simulink model "xe_hai_banh_cb"  (R2019a)
settings: Solver=FixedStepAuto  StartTime=0.0  StopTime=20  FixedStep=0.01  RelTol=1e-3
undefined symbols (not defined in the file): a, beta, fw, J_phi, Jm, Jw, L, M, m, n, R, W, x1_in, x2_in, x4_in, x5_in, x7_in, x8_in
settings Model: Creator=ACER  LastModifiedBy=chute

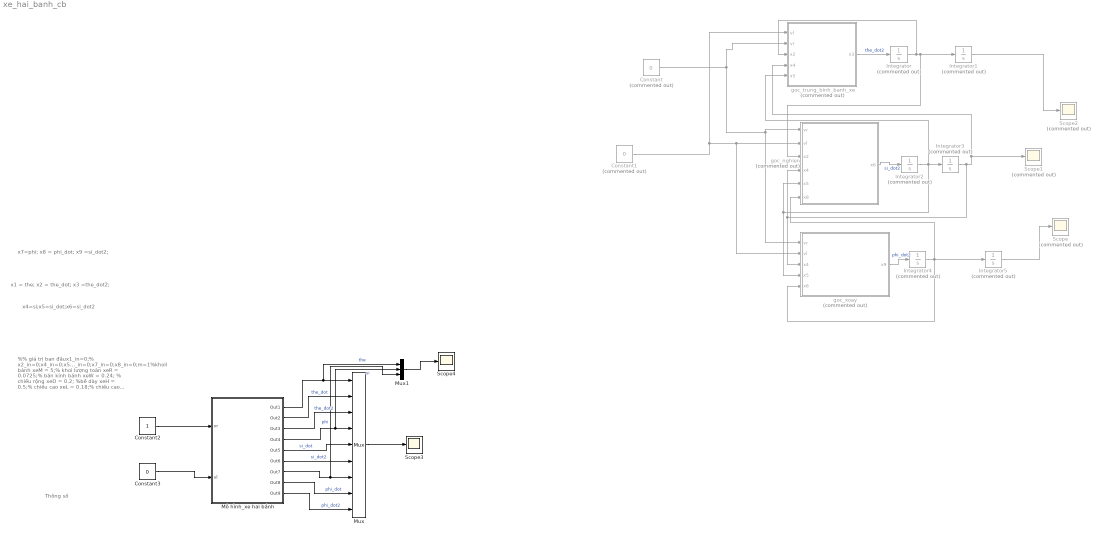
== system xe_hai_banh_cb ==
  note: x4=si;x5=si_dot;x6=si_dot2
  note: %% giá trị ban đầux1_in=0;% x2_in=0;x4_in=0;x5_in=0;x7_in=0;x8_in=0;m=1%khoil bánh xeM = 5;% khoi lượng toàn xeR = 0.0725;% bán kính bánh xeW = 0.24; % chiều rộng xeD = 0.2; %bề dày xeH = 0.5;% chiều cao xeL = 0.18;% chiều cao thân xefw = 0.18;% hệ số ma sát mặt di chuyểnfm = 0.002;% hệ số ma sát động cơJm = m*R^2/2;% momen quán tính đcJsi = M*L^2/3; % momen quan tính phần thân xeJ_phi = M*(W^2 + D^2)/12; % momen quan tinh toàn xeJw = m*R^2/2; %momen quan tinh banh xeRm = 50; % ddien trở Kb = 0.468; % hệ số dcKt = 0.317; % hệ số dcn = 40; % tỉ số truyền dcg = 9.81; %gia tóc ttbeta = (n*Kt*Kb)/Rm + fm;a=(n*Kt)/Rm;
  note: Thông số
  note: x1 = the; x2 = the_dot; x3 =the_dot2;
  note: x7=phi; x8 = phi_dot; x9 =si_dot2;
  Constant : Constant  Commented=on  Value=0
  Constant1 : Constant  Commented=on  Value=0
  Constant2 : Constant
  Constant3 : Constant  Value=0
  Integrator : Integrator  Commented=on
  Integrator1 : Integrator  Commented=on  InitialCondition=0.0012
  Integrator2 : Integrator  Commented=on
  Integrator3 : Integrator  Commented=on  InitialCondition=0.0001
  Integrator4 : Integrator  Commented=on
  Integrator5 : Integrator  Commented=on  InitialCondition=0.0001
  Mux : Mux  Inputs=9
  Mux1 : Mux  Inputs=3
  "Mô hình_xe hai bánh " : Subsystem
  Scope : Scope  Commented=on
  Scope1 : Scope  Commented=on
  Scope2 : Scope  Commented=on
  Scope3 : Scope
  Scope4 : Scope
  goc_nghien : MATLAB Function  Commented=on  TreatAsAtomicUnit=on
  goc_trung_binh_banh_xe : MATLAB Function  Commented=on  TreatAsAtomicUnit=on
  "goc_xoay " : MATLAB Function  Commented=on  TreatAsAtomicUnit=on
  wires:
  Integrator/1 -> goc_nghien/3(x2), Integrator1/1, goc_trung_binh_banh_xe/3(x2)
  Integrator4/1 -> "goc_xoay "/5(x8), Integrator5/1, goc_nghien/6(x8)
  Integrator2/1 -> goc_nghien/5(x5), "goc_xoay "/4(x5), goc_trung_binh_banh_xe/5(x5), Integrator3/1
  Integrator3/1 -> goc_nghien/4(x4), "goc_xoay "/3(x4), goc_trung_binh_banh_xe/4(x4), Scope1/1
  Constant1/1 -> goc_trung_binh_banh_xe/1(vl), "goc_xoay "/2(vl), goc_nghien/2(vl)
  goc_nghien/1(x6) -> Integrator2/1  "si_dot2"
  Constant/1 -> goc_trung_binh_banh_xe/2(vr), "goc_xoay "/1(vr), goc_nghien/1(vr)
  "goc_xoay "/1(x9) -> Integrator4/1  "phi_dot2"
  goc_trung_binh_banh_xe/1(x3) -> Integrator/1  "the_dot2"
  Integrator5/1 -> Scope/1
  Integrator1/1 -> Scope2/1
  Mux/1 -> Scope3/1
  "Mô hình_xe hai bánh "/9(Out9) -> Mux/9  "phi_dot2"
  "Mô hình_xe hai bánh "/8(Out8) -> Mux/8  "phi_dot"
  "Mô hình_xe hai bánh "/7(Out7) -> Mux1/3, Mux/7  "phi"
  "Mô hình_xe hai bánh "/6(Out6) -> Mux/6  "si_dot2"
  "Mô hình_xe hai bánh "/5(Out5) -> Mux/5  "si_dot"
  "Mô hình_xe hai bánh "/4(Out4) -> Mux1/2, Mux/4  "si"
  "Mô hình_xe hai bánh "/3(Out3) -> Mux/3  "the_dot2"
  "Mô hình_xe hai bánh "/2(Out2) -> Mux/2  "the_dot"
  "Mô hình_xe hai bánh "/1(Out1) -> Mux1/1, Mux/1  "the"
  Constant2/1 -> "Mô hình_xe hai bánh "/1("vr ")
  Constant3/1 -> "Mô hình_xe hai bánh "/2("vl ")
  Mux1/1 -> Scope4/1

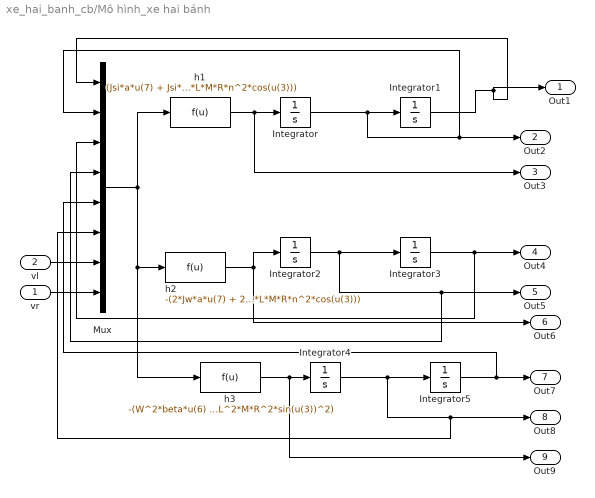
== system xe_hai_banh_cb/Mô hình_xe hai bánh  ==
  "vr " : Inport
  "vl " : Inport  Port=2
  Integrator : Integrator  InitialCondition=x2_in
  Integrator1 : Integrator  InitialCondition=x1_in
  Integrator2 : Integrator  InitialCondition=x5_in
  Integrator3 : Integrator  InitialCondition=x4_in
  Integrator4 : Integrator  InitialCondition=x8_in
  Integrator5 : Integrator  InitialCondition=x7_in
  Mux : Mux  Inputs=8
  "h1 " : Fcn  Expr=(Jsi*a*u(7) + Jsi*a*u(8) - 2*Jsi*beta*u(2) + 2*Jsi*beta*u(4) - 2*Jsi*fw*u(2) + L^2*M*a*u(7) + L^2*M*a*u(8) - 2*L^2*M*beta*u(2) + 2*L^2*M*beta*u(4) - 2*L^2*M*fw*u(2) - 4*Jm*fw*n^2*u(2) + L^3*M^2*R*u(4)^2*sin(u(3)) - 2*L*M*R*beta*u(2)*cos(u(3)) + 2*L*M*R*beta*u(4)*cos(u(3)) - L^3*M^2*R*u(6)^2*cos(u(3))^2*sin(u(3)) - L^2*M^2*R*g*cos(u(3))*sin(u(3)) + Jsi*L*M*R*u(4)^2*sin(u(3)) + 2*Jm*L*M*g*n^2*sin(u(3)) + L*M*R*a*u(7)*cos(u(3)) + L*M*R*a*u(8)*cos(u(3)) + 2*Jm*L^2*M*n^2*u(6)^2*cos(u(3))*sin(u(3)) + 2*Jm*L*M*R*n^2*u(4)^2*sin(u(3)))/(2*Jsi*Jw + L^2*M^2*R^2 + 2*Jw*L^2*M + Jsi*M*R^2 + 2*Jm*Jsi*n^2 + 4*Jm*Jw*n^2 + 2*Jsi*R^2*m + 2*Jm*L^2*M*n^2 + 2*Jm*M*R^2*n^2 + 2*L^2*M*R^2*m + 4*Jm*R^2*m*n^2 - L^2*M^2*R^2*cos(u(3))^2 + 4*Jm*L*M*R*n^2*cos(u(3)))
  "h2 " : Fcn  Expr=-(2*Jw*a*u(7) + 2*Jw*a*u(8) - 4*Jw*beta*u(2) + 4*Jw*beta*u(4) + M*R^2*a*u(7) + M*R^2*a*u(8) - 2*M*R^2*beta*u(2) + 2*M*R^2*beta*u(4) + 2*R^2*a*m*u(7) + 2*R^2*a*m*u(8) + 4*Jm*fw*n^2*u(2) - 4*R^2*beta*m*u(2) + 4*R^2*beta*m*u(4) - L*M^2*R^2*g*sin(u(3)) - 2*Jw*L*M*g*sin(u(3)) - 2*L*M*R*beta*u(2)*cos(u(3)) + 2*L*M*R*beta*u(4)*cos(u(3)) - 2*L*M*R*fw*u(2)*cos(u(3)) + L^2*M^2*R^2*u(4)^2*cos(u(3))*sin(u(3)) - L^2*M^2*R^2*u(6)^2*cos(u(3))*sin(u(3)) - 2*Jw*L^2*M*u(6)^2*cos(u(3))*sin(u(3)) - 2*Jm*L*M*g*n^2*sin(u(3)) - 2*L*M*R^2*g*m*sin(u(3)) + L*M*R*a*u(7)*cos(u(3)) + L*M*R*a*u(8)*cos(u(3)) - 2*Jm*L^2*M*n^2*u(6)^2*cos(u(3))*sin(u(3)) - 2*L^2*M*R^2*m*u(6)^2*cos(u(3))*sin(u(3)) - 2*Jm*L*M*R*n^2*u(4)^2*sin(u(3)))/(2*Jsi*Jw + L^2*M^2*R^2 + 2*Jw*L^2*M + Jsi*M*R^2 + 2*Jm*Jsi*n^2 + 4*Jm*Jw*n^2 + 2*Jsi*R^2*m + 2*Jm*L^2*M*n^2 + 2*Jm*M*R^2*n^2 + 2*L^2*M*R^2*m + 4*Jm*R^2*m*n^2 - L^2*M^2*R^2*cos(u(3))^2 + 4*Jm*L*M*R*n^2*cos(u(3)))
  "h3 " : Fcn  Expr=-(W^2*beta*u(6) + W^2*fw*u(6) + R*W*a*u(7) - R*W*a*u(8) + 4*L^2*M*R^2*u(4)*u(6)*cos(u(3))*sin(u(3)))/(2*J_phi*R^2 + Jw*W^2 + Jm*W^2*n^2 + R^2*W^2*m + 2*L^2*M*R^2*sin(u(3))^2)
  Out1 : Outport
  Out2 : Outport  Port=2
  Out3 : Outport  Port=3
  Out4 : Outport  Port=4
  Out5 : Outport  Port=5
  Out6 : Outport  Port=6
  Out7 : Outport  Port=7
  Out8 : Outport  Port=8
  Out9 : Outport  Port=9
  wires:
  Mux/1 -> "h2 "/1, "h3 "/1, "h1 "/1
  "vr "/1 -> Mux/8
  "vl "/1 -> Mux/7
  Integrator/1 -> Mux/2, Out2/1, Integrator1/1
  Integrator1/1 -> Mux/1, Out1/1
  "h2 "/1 -> Integrator2/1, Out6/1
  "h3 "/1 -> Out9/1, Integrator4/1
  Integrator4/1 -> Mux/6, Out8/1, Integrator5/1
  Integrator3/1 -> Mux/3, Out4/1
  Integrator5/1 -> Mux/5, Out7/1
  "h1 "/1 -> Out3/1, Integrator/1
  Integrator2/1 -> Mux/4, Out5/1, Integrator3/1

== matlab function xe_hai_banh_cb/goc_nghien ==
  data: vr input; x6 output; vl input; x2 input; x4 input; x5 input; x8 input
function x6= si_dot2(vr,vl,x2,x4,x5,x8)
m=1%khoil bánh xe
M = 5;% khoi lượng toàn xe
R = 0.0725;% bán kính bánh xe
W = 0.24; % chiều rộng xe
D = 0.2 %bề dày xe
H = 0.5;% chiều cao xe
L = 0.18;% chiều cao thân xe
fw = 0.18;% hệ số ma sát mặt di chuyển
fm = 0.002;% hệ số ma sát động cơ
Jm = m*R^2/2;% momen quán tính đc
Jsi = M*L^2/3; % momen quan tính phần thân xe
J_phi = M*(W^2 + D^2)/12; % momen quan tinh toàn xe
Jw = m*R^2/2; %momen quan tinh banh xe
Rm = 50; % ddien trở 
Kb = 0.468; % hệ số dc
Kt = 0.317; % hệ số dc
n = 40; % tỉ số truyền dc
g = 9.81; %gia tóc tt
beta = (n*Kt*Kb)/Rm + fm;
a=(n*Kt)/Rm;
x6= -(2*Jw*a*vl + 2*Jw*a*vr - 4*Jw*beta*x2 + ...
    4*Jw*beta*x5 + M*R^2*a*vl + M*R^2*a*vr -...
    2*M*R^2*beta*x2 + 2*M*R^2*beta*x5 + 2*R^2*a*m*vl +...
    2*R^2*a*m*vr + 4*Jm*fw*n^2*x2 - 4*R^2*beta*m*x2 +...
    4*R^2*beta*m*x5 - L*M^2*R^2*g*sin(x4) - 2*Jw*L*M*g*sin(x4) - ...
    2*L*M*R*beta*x2*cos(x4) + 2*L*M*R*beta*x5*cos(x4) - 2*L*M*R*fw*x2*cos(x4) +...
    L^2*M^2*R^2*x5^2*cos(x4)*sin(x4) - L^2*M^2*R^2*x8^2*cos(x4)*sin(x4) -...
    2*Jw*L^2*M*x8^2*cos(x4)*sin(x4) - 2*Jm*L*M*g*n^2*sin(x4) - ...
    2*L*M*R^2*g*m*sin(x4) + L*M*R*a*vl*cos(x4) + L*M*R*a*vr*cos(x4) -...
    2*Jm*L^2*M*n^2*x8^2*cos(x4)*sin(x4) - 2*L^2*M*R^2*m*x8^2*cos(x4)*sin(x4) -...
    2*Jm*L*M*R*n^2*x5^2*sin(x4))/(2*Jsi*Jw + L^2*M^2*R^2 +...
    2*Jw*L^2*M + Jsi*M*R^2 + 2*Jm*Jsi*n^2 + 4*Jm*Jw*n^2 +...
    2*Jsi*R^2*m + 2*Jm*L^2*M*n^2 + 2*Jm*M*R^2*n^2 + 2*L^2*M*R^2*m +...
    4*Jm*R^2*m*n^2 - L^2*M^2*R^2*cos(x4)^2 + 4*Jm*L*M*R*n^2*cos(x4));

== matlab function xe_hai_banh_cb/goc_trung_binh_banh_xe ==
  data: vl input; x3 output; vr input; x2 input; x4 input; x5 input
function x3 =the_dot2(vl,vr,x2,x4,x5)
m=1%khoil bánh xe
M = 5;% khoi lượng toàn xe
R = 0.0725;% bán kính bánh xe
W = 0.24; % chiều rộng xe
D = 0.2 %bề dày xe
H = 0.5;% chiều cao xe
L = 0.18;% chiều cao thân xe
fw = 0.18;% hệ số ma sát mặt di chuyển
fm = 0.002;% hệ số ma sát động cơ
Jm = m*R^2/2;% momen quán tính đc
Jsi = M*L^2/3; % momen quan tính phần thân xe
J_phi = M*(W^2 + D^2)/12; % momen quan tinh toàn xe
Jw = m*R^2/2; %momen quan tinh banh xe
Rm = 50; % ddien trở 
Kb = 0.468; % hệ số dc
Kt = 0.317; % hệ số dc
n = 40; % tỉ số truyền dc
g = 9.81; %gia tóc tt
beta = (n*Kt*Kb)/Rm + fm;
a=(n*Kt)/Rm;
 x3=(Jsi*a*vl + Jsi*a*vr - 2*Jsi*beta*x2 + 2*Jsi*beta*x5 -...
     2*Jsi*fw*x2 + L^2*M*a*vl + L^2*M*a*vr - 2*L^2*M*beta*x2 +...
     2*L^2*M*beta*x5 - 2*L^2*M*fw*x2 - 4*Jm*fw*n^2*x2 +...
     L^3*M^2*R*x5^2*sin(x4) - 2*L*M*R*beta*x2*cos(x4) + 2*L*M*R*beta*x5*cos(x4)...
     - L^3*M^2*R*x8^2*cos(x4)^2*sin(x4) - L^2*M^2*R*g*cos(x4)*sin(x4) +...
     Jsi*L*M*R*x5^2*sin(x4) + 2*Jm*L*M*g*n^2*sin(x4) + L*M*R*a*vl*cos(x4) +...
     L*M*R*a*vr*cos(x4) + 2*Jm*L^2*M*n^2*x8^2*cos(x4)*sin(x4) +...
     2*Jm*L*M*R*n^2*x5^2*sin(x4))/(2*Jsi*Jw + L^2*M^2*R^2 + 2*Jw*L^2*M +...
     Jsi*M*R^2 + 2*Jm*Jsi*n^2 + 4*Jm*Jw*n^2 + 2*Jsi*R^2*m + 2*Jm*L^2*M*n^2 +...
     2*Jm*M*R^2*n^2 + 2*L^2*M*R^2*m + 4*Jm*R^2*m*n^2 - L^2*M^2*R^2*cos(x4)^2 +...
     4*Jm*L*M*R*n^2*cos(x4));
end

== matlab function xe_hai_banh_cb/goc_xoay  ==
  data: vr input; x9 output; vl input; x4 input; x5 input; x8 input
function x9 = phi_dot2(vr,vl,x4,x5,x8)
m=1;%khoil bánh xe
M = 5;% khoi lượng toàn xe
R = 0.0725;% bán kính bánh xe
W = 0.24; % chiều rộng xe
D = 0.2 %bề dày xe
H = 0.5;% chiều cao xe
L = 0.18;% chiều cao thân xe
fw = 0.18;% hệ số ma sát mặt di chuyển
fm = 0.002;% hệ số ma sát động cơ
Jm = m*R^2/2;% momen quán tính đc
Jsi = M*L^2/3; % momen quan tính phần thân xe
J_phi = M*(W^2 + D^2)/12; % momen quan tinh toàn xe
Jw = m*R^2/2; %momen quan tinh banh xe
Rm = 50; % ddien trở 
Kb = 0.468; % hệ số dc
Kt = 0.317; % hệ số dc
n = 40; % tỉ số truyền dc
g = 9.81; %gia tóc tt
beta = (n*Kt*Kb)/Rm + fm;
a=(n*Kt)/Rm;
x9 = -(W^2*beta*x8 + W^2*fw*x8 + R*W*a*vl -...
    R*W*a*vr + 4*L^2*M*R^2*x5*x8*cos(x4)*sin(x4))/(2*J_phi*R^2 +...
    Jw*W^2 + Jm*W^2*n^2 + R^2*W^2*m + 2*L^2*M*R^2*sin(x4)^2);
end
